simulink model "FederMasse"  (R2016a)
settings: Solver=VariableStepAuto  StartTime=0.0  StopTime=tend  RelTol=1e-3
values from neighbouring files (symbols this model uses):
  g = 4^(-2)    (= 0.0625)    [a1.m]    (also in a61.m = 9.81; a62.m = 9.81; a72feder.m = 19.81)
  k = round(2.5)    [a1.m]    (also in a2.m = a.*b; a72feder.m = 10)
  m = round(-1.5)    [a1.m]    (also in a2.m = exp(a); a33.m = 2; a72feder.m = 1)
  r = linspace(0,pi,200)    [a2.m]    (also in a31.m = [ranzen;ranzen;ranzen;ranzen]; a62.m = 3; a72feder.m = 0.3)
  x_0 = 0.3    [a72feder.m]
settings Model: Creator=mam1205  LastModifiedBy=mam1205

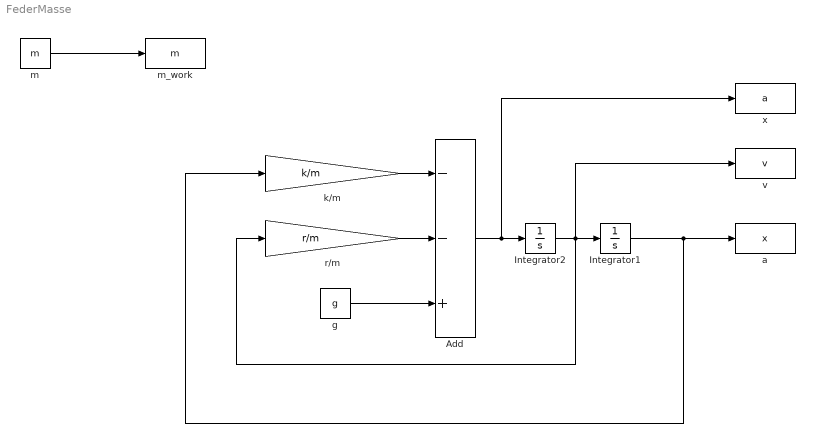
== system FederMasse ==
  Add : Sum  Inputs=--+
  Integrator1 : Integrator  InitialCondition=x_0
      settings: AttributesFormatString=%<InitialCondition>
  Integrator2 : Integrator
      settings: AttributesFormatString=%<InitialCondition>
  a : ToWorkspace  VariableName=x  SaveFormat=Timeseries  SampleTime=-1
  g : Constant  Value=g
  "k/m " : Gain  Gain=k/m
  m : Constant  Value=m
  m_work : ToWorkspace  VariableName=m  SaveFormat=Timeseries  SampleTime=-1
  r/m : Gain  Gain=r/m
  v : ToWorkspace  VariableName=v  SaveFormat=Timeseries  SampleTime=-1
  x : ToWorkspace  VariableName=a  SaveFormat=Timeseries  SampleTime=-1
  wires:
  g/1 -> Add/3
  r/m/1 -> Add/2
  "k/m "/1 -> Add/1
  Add/1 -> x/1, Integrator2/1
  Integrator1/1 -> "k/m "/1, a/1
  m/1 -> m_work/1
  Integrator2/1 -> r/m/1, v/1, Integrator1/1
